simulink model "marble"  (Simulink 4.00)
settings: Solver=ode45  StartTime=0.0  StopTime=20.0  RelTol=1e-3
settings Model: Creator=tjanas  LastModifiedBy=tjanas  ExtModeAutoUpdateStatusClock=off  BooleanDataType=on

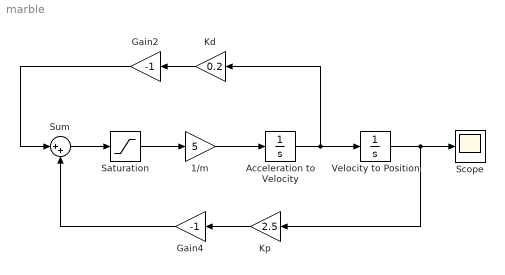
== system marble ==
  1/m : Gain  Gain=5  Multiplication=Element-wise(K.*u)  SaturateOnIntegerOverflow=on
  Acceleration to Velocity : Integrator  ExternalReset=none  InitialConditionSource=internal  InitialCondition=50  LimitOutput=off  UpperSaturationLimit=inf  LowerSaturationLimit=-inf  ShowSaturationPort=off  ShowStatePort=off  AbsoluteTolerance=auto
  Gain2 : Gain  Orientation=left  Gain=-1  Multiplication=Element-wise(K.*u)  SaturateOnIntegerOverflow=on
  Gain4 : Gain  Orientation=left  Gain=-1  Multiplication=Element-wise(K.*u)  SaturateOnIntegerOverflow=on
  Kd : Gain  Orientation=left  Gain=0.2  Multiplication=Element-wise(K.*u)  SaturateOnIntegerOverflow=on
  Kp : Gain  Orientation=left  Gain=2.5  Multiplication=Element-wise(K.*u)  SaturateOnIntegerOverflow=on
  Saturation : Saturate  UpperLimit=5  LowerLimit=-5  LinearizeAsGain=on
  Scope : Scope
      settings: TimeRange=auto  YMin=-5  YMax=5  SaveToWorkspace=off  SaveName=ScopeData  LimitDataPoints=on  MaxDataPoints=5000
  Sum : Sum  Inputs=|++  SaturateOnIntegerOverflow=on
  Velocity to Position : Integrator  ExternalReset=none  InitialConditionSource=internal  InitialCondition=4  LimitOutput=off  UpperSaturationLimit=inf  LowerSaturationLimit=-inf  ShowSaturationPort=off  ShowStatePort=off  AbsoluteTolerance=auto
  wires:
  Kd/1 -> Gain2/1
  1/m/1 -> Acceleration to Velocity/1
  Acceleration to Velocity/1 -> Velocity to Position/1, Kd/1
  Gain2/1 -> Sum/1
  Kp/1 -> Gain4/1
  Gain4/1 -> Sum/2
  Velocity to Position/1 -> Scope/1, Kp/1
  Sum/1 -> Saturation/1
  Saturation/1 -> 1/m/1
